simulink model "RoboticArm"  (R2019b)
settings: Solver=VariableStepAuto  StartTime=0.0  StopTime=10.0  RelTol=1e-3
values from neighbouring files (symbols this model uses):
  F = place(A,B,lambda_desired)    [Code.m]    (also in matlab.mat = [79587.5162501 40579.25 534.36 38])
  I = 1    [Code.m]    (also in matlab.mat)
  J = 1    [Code.m]    (also in matlab.mat)
  k = 0.08    [Code.m]    (also in matlab.mat)
  mgl = 5    [Code.m]    (also in matlab.mat)
  x1ss = pi/3    (= 1.0471975512)    [Code.m]    (also in matlab.mat)
  x2ss = 0    [Code.m]    (also in matlab.mat)
  x4ss = 0    [Code.m]    (also in matlab.mat)
settings Model: Creator=keeyanhaghshenas  LastModifiedBy=keeyanhaghshenas

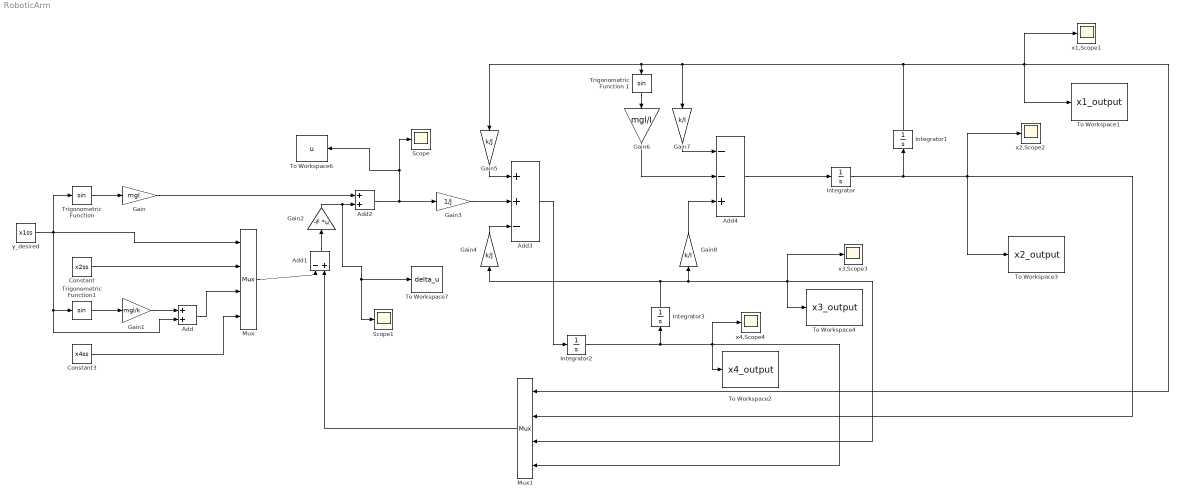
== system RoboticArm ==
  Add : Sum
  Add1 : Sum  Inputs=-+
  Add2 : Sum
  Add3 : Sum  Inputs=++-
  Add4 : Sum  Inputs=--+
  Constant : Constant  Value=x2ss  VectorParams1D=off
  Constant3 : Constant  Value=x4ss  VectorParams1D=off
  Gain : Gain  Gain=mgl
  Gain1 : Gain  Gain=mgl/k
  Gain2 : Gain  Gain=-F  Multiplication=Matrix(K*u)
  Gain3 : Gain  Gain=1/J
  Gain4 : Gain  Gain=k/J
  Gain5 : Gain  Gain=k/J
  Gain6 : Gain  Gain=mgl/I
  Gain7 : Gain  Gain=k/I
  Gain8 : Gain  Gain=k/I
  Integrator{,1..3} (4 alike) : Integrator
  Mux : Mux
  Mux1 : Mux
  Scope : Scope
  Scope1 : Scope
  To Workspace1 : ToWorkspace  VariableName=x1_output  SampleTime=-1
      settings: Save2DSignal=2-D array (concatenate along first dimension)
  To Workspace2 : ToWorkspace  VariableName=x4_output  SampleTime=-1
      settings: Save2DSignal=2-D array (concatenate along first dimension)
  To Workspace3 : ToWorkspace  VariableName=x2_output  SampleTime=-1
      settings: Save2DSignal=2-D array (concatenate along first dimension)
  To Workspace4 : ToWorkspace  VariableName=x3_output  SampleTime=-1
      settings: Save2DSignal=2-D array (concatenate along first dimension)
  To Workspace6 : ToWorkspace  VariableName=u  SampleTime=-1
      settings: Save2DSignal=2-D array (concatenate along first dimension)
  To Workspace7 : ToWorkspace  VariableName=delta_u  SampleTime=-1
      settings: Save2DSignal=2-D array (concatenate along first dimension)
  "Trigonometric Function " : Trigonometry
  Trigonometric Function 1 : Trigonometry
  Trigonometric Function1 : Trigonometry
  x1,Scope1 : Scope
  x2,Scope2 : Scope
  x3,Scope3 : Scope
  x4,Scope4 : Scope
  "y_desired " : Constant  Value=x1ss
  wires:
  "y_desired "/1 -> Mux/1, Trigonometric Function1/1, Add/2, "Trigonometric Function "/1
  "Trigonometric Function "/1 -> Gain/1
  Trigonometric Function1/1 -> Gain1/1
  Constant/1 -> Mux/2
  Gain1/1 -> Add/1
  Add/1 -> Mux/3
  Constant3/1 -> Mux/4
  Mux/1 -> Add1/1
  Add1/1 -> Gain2/1
  Gain2/1 -> Scope1/1, To Workspace7/1, Add2/2
  Gain/1 -> Add2/1
  Add2/1 -> To Workspace6/1, Scope/1, Gain3/1
  Gain3/1 -> Add3/2
  Gain5/1 -> Add3/1
  Gain4/1 -> Add3/3
  Trigonometric Function 1/1 -> Gain6/1
  Gain6/1 -> Add4/2
  Gain7/1 -> Add4/1
  Mux1/1 -> Add1/2
  Add4/1 -> Integrator/1
  Integrator1/1 -> Gain7/1, Gain5/1, Trigonometric Function 1/1, To Workspace1/1, x1,Scope1/1, Mux1/1
  Integrator/1 -> To Workspace3/1, Mux1/2, x2,Scope2/1, Integrator1/1
  Add3/1 -> Integrator2/1
  Integrator2/1 -> Integrator3/1, To Workspace2/1, x4,Scope4/1, Mux1/4
  Integrator3/1 -> Gain8/1, To Workspace4/1, x3,Scope3/1, Mux1/3, Gain4/1
  Gain8/1 -> Add4/3
